simulink model "MCU_LuenbergerObserver_dsPIC33AK128MC106"  (R2024a)
settings: Solver=FixedStepDiscrete  StartTime=0.0  StopTime=inf  FixedStep=50e-6  RelTol=1e-3  EnableMultiTasking=on
undefined symbols (not defined in the file or in its folder): A0, A4, ADC, B0, C10, C11, C6, C7, C8, control, D11, D12, DiscIntNeverNeededParam, inverter, Max, MaxPer, motor, ms, NumBits1, NumBits2, P1, P17, P20, P39, P40, P41, P43, P44, P60, P61, Pin, PosRange1, PosRange2, PWM1_Trg1, Resol, s, Slope1, Slope2, us
libraries: simulink x34, MCHP_Blockset x18
(part 5 of 5)

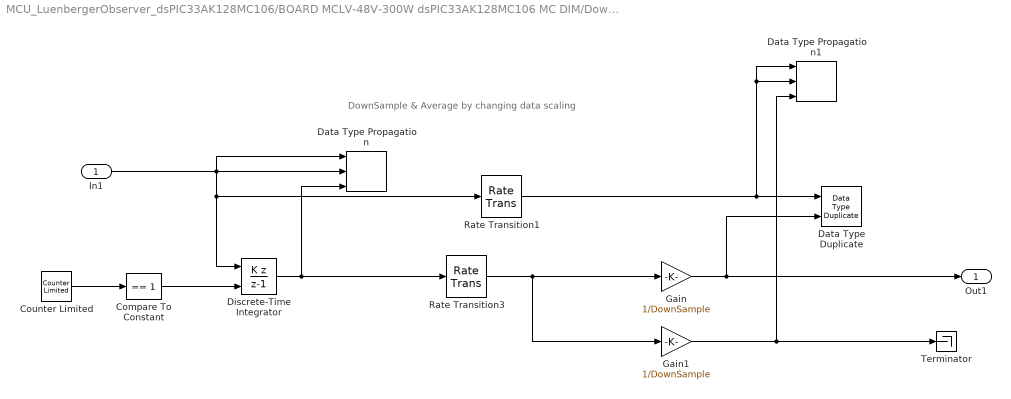
== system MCU_LuenbergerObserver_dsPIC33AK128MC106/BOARD MCLV-48V-300W dsPIC33AK128MC106 MC DIM/Downsample x20 ==
  note: DownSample & Average by changing data scaling
  In1 : Inport
  Compare To Constant : simulink/Logic and Bit Operations/Compare To Constant  relop===  const=1  OutDataTypeStr=boolean
  Counter Limited : simulink/Sources/Counter Limited  uplimit=DownSample-1  tsamp=-1
  Data Type Duplicate : DataTypeDuplicate
  Data Type Propagation : simulink/Signal Attributes/Data Type Propagation  PropDataType=fixdt(1, 16)  IfRefDouble=double  IfRefSingle=single  IsSigned=IsSigned1 or IsSigned2  NumBitsBase=NumBits1+NumBits2  NumBitsMult=1  NumBitsAdd=0  NumBitsAllowFinal=1:128  PropScaling=2^-10  ValuesUsedBestPrec=[5 -7]  SlopeBase=Slope1  SlopeMult=1  SlopeAdd=0  BiasBase=Bias1  BiasMult=1  BiasAdd=0
  Data Type Propagation1 : simulink/Signal Attributes/Data Type Propagation  PropDataType=fixdt(1, 16)  IfRefDouble=double  IfRefSingle=single  IsSigned=IsSigned1 or IsSigned2  NumBitsBase=NumBits1+NumBits2  NumBitsMult=1  NumBitsAdd=0  NumBitsAllowFinal=1:128  PropScaling=2^-10  ValuesUsedBestPrec=[5 -7]  SlopeBase=PosRange1  SlopeMult=1  SlopeAdd=0  BiasBase=Bias1  BiasMult=1  BiasAdd=0
  Discrete-Time Integrator : DiscreteIntegrator  IntegratorMethod=Accumulation: Backward Euler  gainval=1  ExternalReset=sampled level  SampleTime=-1  OutDataTypeStr=Inherit: Inherit via back propagation  ICPrevOutput=DiscIntNeverNeededParam  ICPrevScaledInput=DiscIntNeverNeededParam
  Gain : Gain  Gain=1/DownSample  OutDataTypeStr=Inherit: Inherit via back propagation  RndMeth=Round
  Gain1 : Gain  Gain=1/DownSample  OutDataTypeStr=Inherit: Inherit via back propagation
  Rate Transition1 : RateTransition  OutPortSampleTimeOpt=Multiple of input port sample time  OutPortSampleTimeMultiple=DownSample  OutPortSampleTime=DownSample
  Rate Transition3 : RateTransition  OutPortSampleTimeOpt=Multiple of input port sample time  OutPortSampleTimeMultiple=DownSample  OutPortSampleTime=DownSample
  Terminator : Terminator
  Out1 : Outport  VectorParamsAs1DForOutWhenUnconnected=off
  wires:
  Gain1/1 -> Data Type Propagation1/3, Terminator/1
  Rate Transition1/1 -> Data Type Duplicate/1, Data Type Propagation1/1, Data Type Propagation1/2
  Gain/1 -> Out1/1, Data Type Duplicate/2
  Counter Limited/1 -> Compare To Constant/1
  Discrete-Time Integrator/1 -> Rate Transition3/1, Data Type Propagation/3
  Compare To Constant/1 -> Discrete-Time Integrator/2
  In1/1 -> Data Type Propagation/1, Data Type Propagation/2, Discrete-Time Integrator/1, Rate Transition1/1
  Rate Transition3/1 -> Gain/1, Gain1/1

== system MCU_LuenbergerObserver_dsPIC33AK128MC106/BOARD MCLV-48V-300W dsPIC33AK128MC106 MC DIM/Downsample x20 _ ==
  note: DownSample & Average by changing data scaling
  In1 : Inport
  Compare To Constant : simulink/Logic and Bit Operations/Compare To Constant  relop===  const=1  OutDataTypeStr=boolean
  Counter Limited : simulink/Sources/Counter Limited  uplimit=DownSample-1  tsamp=-1
  Data Type Duplicate : DataTypeDuplicate
  Data Type Propagation : simulink/Signal Attributes/Data Type Propagation  PropDataType=fixdt(1, 16)  IfRefDouble=double  IfRefSingle=single  IsSigned=IsSigned1 or IsSigned2  NumBitsBase=NumBits1+NumBits2  NumBitsMult=1  NumBitsAdd=0  NumBitsAllowFinal=1:128  PropScaling=2^-10  ValuesUsedBestPrec=[5 -7]  SlopeBase=Slope1  SlopeMult=1  SlopeAdd=0  BiasBase=Bias1  BiasMult=1  BiasAdd=0
  Data Type Propagation1 : simulink/Signal Attributes/Data Type Propagation  PropDataType=fixdt(1, 16)  IfRefDouble=double  IfRefSingle=single  IsSigned=IsSigned1 or IsSigned2  NumBitsBase=NumBits1+NumBits2  NumBitsMult=1  NumBitsAdd=0  NumBitsAllowFinal=1:128  PropScaling=2^-10  ValuesUsedBestPrec=[5 -7]  SlopeBase=PosRange1  SlopeMult=1  SlopeAdd=0  BiasBase=Bias1  BiasMult=1  BiasAdd=0
  Discrete-Time Integrator : DiscreteIntegrator  IntegratorMethod=Accumulation: Backward Euler  gainval=1  ExternalReset=sampled level  SampleTime=-1  OutDataTypeStr=Inherit: Inherit via back propagation  ICPrevOutput=DiscIntNeverNeededParam  ICPrevScaledInput=DiscIntNeverNeededParam
  Gain : Gain  Gain=1/DownSample  OutDataTypeStr=Inherit: Inherit via back propagation  RndMeth=Round
  Gain1 : Gain  Gain=1/DownSample  OutDataTypeStr=Inherit: Inherit via back propagation
  Rate Transition1 : RateTransition  OutPortSampleTimeOpt=Multiple of input port sample time  OutPortSampleTimeMultiple=DownSample  OutPortSampleTime=DownSample
  Rate Transition3 : RateTransition  OutPortSampleTimeOpt=Multiple of input port sample time  OutPortSampleTimeMultiple=DownSample  OutPortSampleTime=DownSample
  Terminator : Terminator
  Out1 : Outport  VectorParamsAs1DForOutWhenUnconnected=off
  wires:
  Rate Transition3/1 -> Gain1/1, Gain/1
  In1/1 -> Rate Transition1/1, Discrete-Time Integrator/1, Data Type Propagation/2, Data Type Propagation/1
  Compare To Constant/1 -> Discrete-Time Integrator/2
  Discrete-Time Integrator/1 -> Data Type Propagation/3, Rate Transition3/1
  Counter Limited/1 -> Compare To Constant/1
  Gain/1 -> Data Type Duplicate/2, Out1/1
  Rate Transition1/1 -> Data Type Propagation1/2, Data Type Propagation1/1, Data Type Duplicate/1
  Gain1/1 -> Terminator/1, Data Type Propagation1/3

== system MCU_LuenbergerObserver_dsPIC33AK128MC106/BOARD MCLV-48V-300W dsPIC33AK128MC106 MC DIM/MCLV 48V-300W board webpage ==

== system MCU_LuenbergerObserver_dsPIC33AK128MC106/BOARD MCLV-48V-300W dsPIC33AK128MC106 MC DIM/Timing Analysis ==
  note: CPU overload is 0 if no overload took place between two MCU Overload block execution.
      | Otherwise, bits field output code for TID(s) responsible for at least one overload.
  Downsample Averaged2 : Subsystem  mask{InputSampleTime=.0005, DownSample=200}
      mask prompts: InputSampleTime "Input sample time"; DownSample "DownSample Factor"
  Gain : Gain  Gain=5e-9/.0005 * 100  OutMin=0  OutMax=100  OutDataTypeStr=fixdt(0,16)  RndMeth=Simplest  SaturateOnIntegerOverflow=on
  MCU Load : MCHP_Blockset/Profiling/MCU Load  MCULoadPin_TXT=None  MCULoadMeasure=on  TIMER_Resolution_TXT="Resol: 0.005(us)  -  Max: 0.328(ms)"  MCHP_TIMER_REQUEST={MCU_Load}{MCU_Load}21:5:0:0:[]:32768;  MCHP_TIMER_RESULT=[2 65535 ]  MCHP_MASTERLINK=MCU_LuenbergerObserver_dsPIC33AK128MC106/BOARD MCLV-48V-300W dsPIC33AK128MC106 MC DIM/Microchip Master  MCHP_COMPILED_INFO="CompiledSampleTime= [0.00050000000000000001041   0 ];CompiledInportDataTypes=[    ];CompiledInportDataWidth=[];"  Info="Timer 2:  Resol: 5(ns)  -  Max: 327.68(us)"  SampleTime=.0005
      settings: SourceProductName=MPLAB Device Blocks for Simulink
  MCU Overload : MCHP_Blockset/Profiling/MCU Overload  MCUOverloadBlockOutput=on  MCUOverLoadPin_TXT=None  MCHP_MASTERLINK=MCU_LuenbergerObserver_dsPIC33AK128MC106/BOARD MCLV-48V-300W dsPIC33AK128MC106 MC DIM/Microchip Master  SampleTime=-1
      settings: SourceProductName=MPLAB Device Blocks for Simulink
  Overload : Constant  Value=65535  OutDataTypeStr=Inherit: Inherit via back propagation
  Rate Transition : RateTransition  Deterministic=off  OutPortSampleTime=.0005*200
  Switch : Switch  Criteria=u2 ~= 0  SaturateOnIntegerOverflow=off  InputSameDT=off
  CPU Load : Outport  Unit=%  SampleTime=.0005*200
  CPU Overload : Outport  Port=2
  wires:
  Gain/1 -> CPU Load/1
  Overload/1 -> Switch/1
  Switch/1 -> Gain/1
  Downsample Averaged2/1(Out1) -> Switch/3
  MCU Load/1 -> Downsample Averaged2/1(In1)
  MCU Overload/1 -> CPU Overload/1, Rate Transition/1
  Rate Transition/1 -> Switch/2

== system MCU_LuenbergerObserver_dsPIC33AK128MC106/Control law/BO ==
  vdqr : Inport
  Enable : EnablePort
  vdq : Outport  VectorParamsAs1DForOutWhenUnconnected=off
  wires:
  vdqr/1 -> vdq/1

== system MCU_LuenbergerObserver_dsPIC33AK128MC106/Control law/Current Control ==
  idq : Inport
  idqr : Inport  Port=2
  om : Inport  Port=3
  gainElec : Inport  Port=4
  Enable : EnablePort  StatesWhenEnabling=reset
  Constant : Constant  Value=motor.p  OutDataTypeStr=single
  Constant1 : Constant  Value=motor.L  OutDataTypeStr=single
  Constant2 : Constant  Value=motor.Phif  OutDataTypeStr=single
  Current : Subsystem
  Voltage Saturation : Subsystem
  feedback lineazation : Subsystem
  v_dq : Outport
  wires:
  Constant1/1 -> feedback lineazation/5(L)
  Constant2/1 -> feedback lineazation/6(Phif)
  Constant/1 -> feedback lineazation/4(p)
  feedback lineazation/1(v_dq) -> Voltage Saturation/1(vdq)
  Voltage Saturation/2(saturation) -> Current/3(saturation)
  gainElec/1 -> Current/4(Ke)
  idq/1 -> Current/1(idq), feedback lineazation/2(idq)
  Current/1(v_dq) -> feedback lineazation/1(udq)
  idqr/1 -> Current/2(iqr)
  Voltage Saturation/1(vdqsat) -> v_dq/1
  om/1 -> feedback lineazation/3(om)

== system MCU_LuenbergerObserver_dsPIC33AK128MC106/Control law/Mechnical Control ==
  idqr : Inport
  om : Inport  Port=2
  omr : Inport  Port=3
  gainMeca : Inport  Port=4
  tauest : Inport  Port=5
  Enable : EnablePort  StatesWhenEnabling=reset
  Augmented state feedback : Subsystem
  Mux : Mux  Inputs=2
  Selector : Selector  InputPortWidth=2  IndexOptions=Index vector (dialog)  Indices=1  OutputSizes=1
  idqro : Outport  VectorParamsAs1DForOutWhenUnconnected=off
  wires:
  Selector/1 -> Mux/1
  Mux/1 -> idqro/1
  idqr/1 -> Selector/1
  gainMeca/1 -> Augmented state feedback/3(gainMeca)
  omr/1 -> Augmented state feedback/1(omref)
  Augmented state feedback/1(iqref) -> Mux/2
  om/1 -> Augmented state feedback/2(om)
  tauest/1 -> Augmented state feedback/4(tauest)

== system MCU_LuenbergerObserver_dsPIC33AK128MC106/Control law/Subsystem ==
  idqr : Inport
  Enable : EnablePort
  idqro : Outport
  wires:
  idqr/1 -> idqro/1

== system MCU_LuenbergerObserver_dsPIC33AK128MC106/Control law/off ==
  Enable : EnablePort
  Mux : Mux  Inputs=2
  vd : Constant  Value=0  OutDataTypeStr=single
  vq : Constant  Value=0  OutDataTypeStr=single
  vdq : Outport  VectorParamsAs1DForOutWhenUnconnected=off
  wires:
  vq/1 -> Mux/2
  Mux/1 -> vdq/1
  vd/1 -> Mux/1

== system MCU_LuenbergerObserver_dsPIC33AK128MC106/Init Enc/Wait 1s ==
  Enable : EnablePort  StatesWhenEnabling=reset
  AND : Logic  IconShape=distinctive  AllPortsSameDT=off  OutDataTypeStr=boolean
  Compare To Constant : simulink/Logic and Bit Operations/Compare To Constant  relop=>  const=0.5  OutDataTypeStr=boolean
  Compare To Constant1 : simulink/Logic and Bit Operations/Compare To Constant  relop=>  const=0.6  OutDataTypeStr=boolean
  Constant1 : Constant  OutDataTypeStr=int16
  Discrete-Time Integrator : DiscreteIntegrator  SampleTime=-1  OutDataTypeStr=fixdt(1,32,20)  SaturateOnIntegerOverflow=on  LimitOutput=on  UpperSaturationLimit=2  LowerSaturationLimit=0  ICPrevOutput=DiscIntNeverNeededParam  ICPrevScaledInput=DiscIntNeverNeededParam
  NOT : Logic  Operator=NOT  IconShape=distinctive  AllPortsSameDT=off  OutDataTypeStr=boolean
  init enc : Outport
  init done : Outport  Port=2
  wires:
  Compare To Constant/1 -> AND/1
  Constant1/1 -> Discrete-Time Integrator/1
  Discrete-Time Integrator/1 -> Compare To Constant1/1, Compare To Constant/1
  Compare To Constant1/1 -> init done/1, NOT/1
  AND/1 -> init enc/1
  NOT/1 -> AND/2

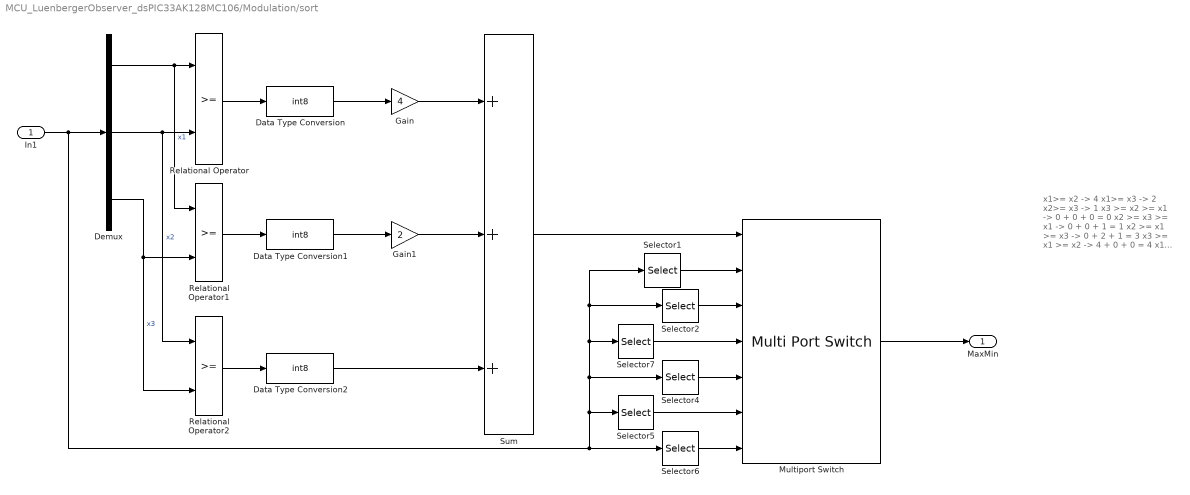
== system MCU_LuenbergerObserver_dsPIC33AK128MC106/Modulation/sort ==
  note: x1>= x2 -> 4
      | x1>= x3 -> 2
      | x2>= x3 -> 1
      |
      | x3 >= x2 >= x1 -> 0 + 0 + 0 = 0
      | x2 >= x3 >= x1 -> 0 + 0 + 1 = 1
      | x2 >= x1 >= x3 -> 0 + 2 + 1 = 3
      | x3 >= x1 >= x2 -> 4 + 0 + 0 = 4
      | x1 >= x3 >= x2 -> 4 + 2 + 0 = 6
      | x1 >= x2 >= x3 -> 4 + 2 + 1 = 7
  In1 : Inport
  Data Type Conversion : DataTypeConversion  OutDataTypeStr=int8  SaturateOnIntegerOverflow=off  RndMeth=Floor
  Data Type Conversion1 : DataTypeConversion  OutDataTypeStr=int8  SaturateOnIntegerOverflow=off  RndMeth=Floor
  Data Type Conversion2 : DataTypeConversion  OutDataTypeStr=int8  SaturateOnIntegerOverflow=off  RndMeth=Floor
  Demux : Demux  Outputs=3
  Gain : Gain  Gain=4  OutDataTypeStr=Inherit: Same as input
  Gain1 : Gain  Gain=2  OutDataTypeStr=Inherit: Same as input
  Multiport Switch : MultiPortSwitch  DataPortOrder=Specify indices  DataPortIndices={0,1,3,4,6,7}  SaturateOnIntegerOverflow=off  InputSameDT=off
  Relational Operator : RelationalOperator  OutDataTypeStr=boolean  RndMeth=Simplest  InputSameDT=off
  Relational Operator1 : RelationalOperator  OutDataTypeStr=boolean  RndMeth=Simplest  InputSameDT=off
  Relational Operator2 : RelationalOperator  OutDataTypeStr=boolean  RndMeth=Simplest  InputSameDT=off
  Selector1 : Selector  InputPortWidth=3  IndexOptions=Index vector (dialog)  Indices=[3 1]  OutputSizes=1
  Selector2 : Selector  InputPortWidth=3  IndexOptions=Index vector (dialog)  Indices=[2 1]  OutputSizes=1
  Selector4 : Selector  InputPortWidth=3  IndexOptions=Index vector (dialog)  Indices=[3 2]  OutputSizes=1
  Selector5 : Selector  InputPortWidth=3  IndexOptions=Index vector (dialog)  Indices=[1 2]  OutputSizes=1
  Selector6 : Selector  InputPortWidth=3  IndexOptions=Index vector (dialog)  Indices=[1 3]  OutputSizes=1
  Selector7 : Selector  InputPortWidth=3  IndexOptions=Index vector (dialog)  Indices=[2 3]  OutputSizes=1
  Sum : Sum  Inputs=+++
  MaxMin : Outport
  wires:
  Multiport Switch/1 -> MaxMin/1
  Selector2/1 -> Multiport Switch/3
  Selector7/1 -> Multiport Switch/4
  Selector4/1 -> Multiport Switch/5
  Selector5/1 -> Multiport Switch/6
  Selector6/1 -> Multiport Switch/7
  Selector1/1 -> Multiport Switch/2
  Sum/1 -> Multiport Switch/1
  Data Type Conversion2/1 -> Sum/3
  Gain/1 -> Sum/1
  Gain1/1 -> Sum/2
  Data Type Conversion1/1 -> Gain1/1
  Data Type Conversion/1 -> Gain/1
  Relational Operator/1 -> Data Type Conversion/1
  Relational Operator1/1 -> Data Type Conversion1/1
  Relational Operator2/1 -> Data Type Conversion2/1
  In1/1 -> Demux/1, Selector6/1, Selector5/1, Selector1/1, Selector2/1, Selector7/1, Selector4/1
  Demux/1 -> Relational Operator/1, Relational Operator1/1  "x1"
  Demux/2 -> Relational Operator/2, Relational Operator2/1  "x2"
  Demux/3 -> Relational Operator1/2, Relational Operator2/2  "x3"

== system MCU_LuenbergerObserver_dsPIC33AK128MC106/Park/Clarke ==
  note: Clark transform
      | $x_{\alpha\beta} = \frac{2}{3}\underbrace{\left[\begin{array}{ccc}1&-\frac{1}{2}&-\frac{1}{2}\\0&\frac{\sqrt{3}}{2}&-\frac{\sqrt{3}}{2}\end{array}\right]}_{C_{23}}x_{abc}$
      | if only 2 currents are measured since $x_a+x_b+x_c = 0$
      | $x_{abc} = \left[\begin{array}{cc}1 & 0\\0 & 1\\-1&-1\end{array}\right]x_{ab}$
      | leading to
      | $x_{\alpha\beta} = \underbrace{\left[\begin{array}{cc}1&0\\\frac{1}{\sqrt{3}}&\frac{2}{\sqrt{3}}\end{array}\right]}_{C_{22}}x_{ab}$
  xab(c) : Inport
  C1 : Gain  Gain=[1/sqrt(3) 2/sqrt(3)]  Multiplication=Matrix(K*u)  OutDataTypeStr=Inherit: Same as input
  Mux : Mux  Inputs=2
  Selector : Selector  InputPortWidth=2  IndexOptions=Index vector (dialog)  Indices=[1]  OutputSizes=1
  xalphabeta : Outport  VectorParamsAs1DForOutWhenUnconnected=off
  wires:
  xab(c)/1 -> Selector/1, C1/1
  Mux/1 -> xalphabeta/1
  Selector/1 -> Mux/1
  C1/1 -> Mux/2

== system MCU_LuenbergerObserver_dsPIC33AK128MC106/Park/Park ==
  note: Park
      | $x_{dq} = P(\theta)^{-1}x_{\alpha\beta}\\ P(p\theta)^{-1} = \left[\begin{array}{cc}\cos(p\theta) & \sin(p\theta)\\ -\sin(p\theta) & \cos(p\theta) \end{array}\right]$
  xalphabeta : Inport  PortDimensions=2
  P(pth) : Inport  Port=2
  Data Type Duplicate2 : DataTypeDuplicate
  Park : Product  Multiplication=Matrix(*)  OutDataTypeStr=Inherit: Inherit via back propagation  RndMeth=Round
  xdq : Outport  VectorParamsAs1DForOutWhenUnconnected=off
  wires:
  Park/1 -> Data Type Duplicate2/1, xdq/1
  xalphabeta/1 -> Data Type Duplicate2/2, Park/2
  P(pth)/1 -> Park/1

== system MCU_LuenbergerObserver_dsPIC33AK128MC106/Park inverse/Clarke Inverse ==
  note: Clarke inverse
  xalphabeta : Inport
  C23' : Gain  Gain=|  Multiplication=Matrix(K*u)  OutDataTypeStr=Inherit: Inherit via back propagation  RndMeth=Round
      | [1   -1/2        -1/2;
      |         0   sqrt(3)/2   -sqrt(3)/2]'
  xabc : Outport  VectorParamsAs1DForOutWhenUnconnected=off
  wires:
  C23'/1 -> xabc/1
  xalphabeta/1 -> C23'/1

== system MCU_LuenbergerObserver_dsPIC33AK128MC106/Park inverse/Park inverse ==
  note: Inverse Park
      | $x_{\alpha\beta} = P(p\theta)x_{dq}\\ P(p\theta) = \left[\begin{array}{cc}\cos(p\theta) & -\sin(p\theta)\\ \sin(p\theta) & \cos(p\theta) \end{array}\right]$
  xdq : Inport
  P(pth) : Inport  Port=2
  Data Type Duplicate2 : DataTypeDuplicate
  Transpose : Math  Operator=transpose
  Transpose1 : Math  Operator=transpose
  xalpha sin(pth)1 : Product  Multiplication=Matrix(*)  OutDataTypeStr=Inherit: Inherit via back propagation  RndMeth=Round
  xalpahbeta : Outport  VectorParamsAs1DForOutWhenUnconnected=off
  wires:
  xalpha sin(pth)1/1 -> Transpose1/1, Data Type Duplicate2/1
  xdq/1 -> Transpose/1
  Transpose/1 -> xalpha sin(pth)1/1, Data Type Duplicate2/2
  Transpose1/1 -> xalpahbeta/1
  P(pth)/1 -> xalpha sin(pth)1/2

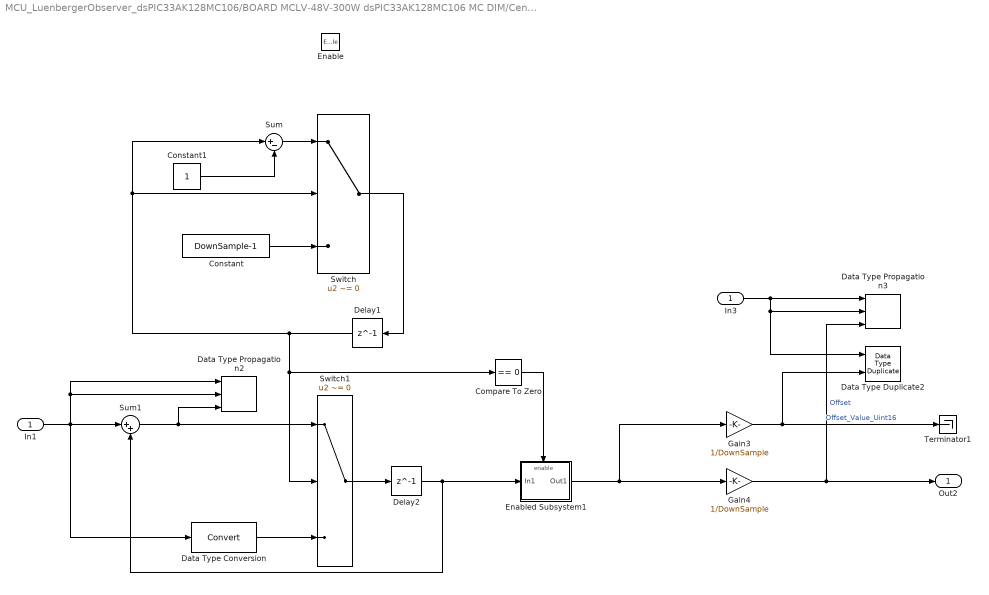
== system MCU_LuenbergerObserver_dsPIC33AK128MC106/BOARD MCLV-48V-300W dsPIC33AK128MC106 MC DIM/Center & sign reversal3/Moving Average ==
  In1 : Inport
  Enable : EnablePort  ZeroCross=off
  Compare To Zero : simulink/Logic and Bit Operations/Compare To Zero  relop===  OutDataTypeStr=boolean
  Constant : Constant  Value=DownSample-1  OutDataTypeStr=uint16
  Constant1 : Constant  OutDataTypeStr=uint16
  Data Type Duplicate2 : DataTypeDuplicate
  Data Type Propagation2 : simulink/Signal Attributes/Data Type Propagation  PropDataType=fixdt(1, 16)  IfRefDouble=double  IfRefSingle=single  IsSigned=IsSigned1 or IsSigned2  NumBitsBase=NumBits1+NumBits2  NumBitsMult=1  NumBitsAdd=0  NumBitsAllowFinal=1:128  PropScaling=2^-10  ValuesUsedBestPrec=[5 -7]  SlopeBase=Slope1  SlopeMult=1  SlopeAdd=0  BiasBase=Bias1  BiasMult=1  BiasAdd=0
  Data Type Propagation3 : simulink/Signal Attributes/Data Type Propagation  PropDataType=fixdt(1, 16)  IfRefDouble=double  IfRefSingle=single  IsSigned=IsSigned1 or IsSigned2  NumBitsBase=NumBits1+NumBits2  NumBitsMult=1  NumBitsAdd=0  NumBitsAllowFinal=1:128  PropScaling=2^-10  ValuesUsedBestPrec=[5 -7]  SlopeBase=PosRange1  SlopeMult=1  SlopeAdd=0  BiasBase=Bias1  BiasMult=1  BiasAdd=0
  Data Type Conversion : DataTypeConversion  SaturateOnIntegerOverflow=off  RndMeth=Floor
  Delay1 : Delay  DelayLength=1  InitialCondition=0
  Delay2 : Delay  DelayLength=1  InitialCondition=[InitialValue * DownSample]
  Enabled Subsystem1 : Subsystem  TreatAsAtomicUnit=on
  Gain3 : Gain  Gain=1/DownSample  OutDataTypeStr=Inherit: Inherit via back propagation  RndMeth=Round
  Gain4 : Gain  Gain=1/DownSample  OutDataTypeStr=Inherit: Inherit via back propagation
  In3 : InportShadow
  Sum : Sum  Inputs=|+-  InputSameDT=on  OutDataTypeStr=Inherit: Same as first input
  Sum1 : Sum  Inputs=|++
  Switch : Switch  Criteria=u2 ~= 0  Threshold=DownSample-1  SaturateOnIntegerOverflow=off  InputSameDT=off
  Switch1 : Switch  Criteria=u2 ~= 0  Threshold=DownSample-1  SaturateOnIntegerOverflow=off
  Terminator1 : Terminator
  Out2 : Outport  InitialOutput=[InitialValue]  VectorParamsAs1DForOutWhenUnconnected=off
  wires:
  Data Type Conversion/1 -> Switch1/3
  In3/1 -> Data Type Propagation3/1, Data Type Propagation3/2, Data Type Duplicate2/1
  Gain4/1 -> Data Type Propagation3/3, Out2/1  "Offset"
  Enabled Subsystem1/1(Out1) -> Gain3/1, Gain4/1
  Gain3/1 -> Terminator1/1, Data Type Duplicate2/2  "Offset_Value_Uint16"
  Compare To Zero/1 -> Enabled Subsystem1/Enable
  Switch1/1 -> Delay2/1
  Sum1/1 -> Switch1/1, Data Type Propagation2/3
  In1/1 -> Sum1/1, Data Type Propagation2/1, Data Type Propagation2/2, Data Type Conversion/1
  Delay2/1 -> Enabled Subsystem1/1(In1), Sum1/2
  Delay1/1 -> Compare To Zero/1, Switch1/2, Sum/1, Switch/2
  Constant/1 -> Switch/3
  Constant1/1 -> Sum/2
  Sum/1 -> Switch/1
  Switch/1 -> Delay1/1

== system MCU_LuenbergerObserver_dsPIC33AK128MC106/BOARD MCLV-48V-300W dsPIC33AK128MC106 MC DIM/Timing Analysis/Downsample Averaged2 ==
  note: DownSample & Average by changing data scaling
  In1 : Inport
  Compare To Constant : simulink/Logic and Bit Operations/Compare To Constant  relop===  const=1  OutDataTypeStr=boolean
  Counter Limited : simulink/Sources/Counter Limited  uplimit=DownSample-1  tsamp=-1
  Data Type Duplicate : DataTypeDuplicate
  Data Type Propagation : simulink/Signal Attributes/Data Type Propagation  PropDataType=fixdt(1, 16)  IfRefDouble=double  IfRefSingle=single  IsSigned=IsSigned1 or IsSigned2  NumBitsBase=NumBits1+NumBits2  NumBitsMult=1  NumBitsAdd=0  NumBitsAllowFinal=1:128  PropScaling=2^-10  ValuesUsedBestPrec=[5 -7]  SlopeBase=Slope1  SlopeMult=1  SlopeAdd=0  BiasBase=Bias1  BiasMult=1  BiasAdd=0
  Data Type Propagation1 : simulink/Signal Attributes/Data Type Propagation  PropDataType=fixdt(1, 16)  IfRefDouble=double  IfRefSingle=single  IsSigned=IsSigned1 or IsSigned2  NumBitsBase=NumBits1+NumBits2  NumBitsMult=1  NumBitsAdd=0  NumBitsAllowFinal=1:128  PropScaling=2^-10  ValuesUsedBestPrec=[5 -7]  SlopeBase=PosRange1  SlopeMult=1  SlopeAdd=0  BiasBase=Bias1  BiasMult=1  BiasAdd=0
  Discrete-Time Integrator : DiscreteIntegrator  IntegratorMethod=Accumulation: Backward Euler  gainval=1  ExternalReset=sampled level  SampleTime=-1  OutDataTypeStr=Inherit: Inherit via back propagation  ICPrevOutput=DiscIntNeverNeededParam  ICPrevScaledInput=DiscIntNeverNeededParam
  Gain : Gain  Gain=1/DownSample  OutDataTypeStr=Inherit: Inherit via back propagation
  Gain1 : Gain  Gain=1/DownSample  OutDataTypeStr=Inherit: Inherit via back propagation
  Rate Transition1 : RateTransition  Deterministic=off  OutPortSampleTime=[InputSampleTime * DownSample]
  Rate Transition3 : RateTransition  OutPortSampleTime=[InputSampleTime * DownSample]
  Terminator : Terminator
  Out1 : Outport  VectorParamsAs1DForOutWhenUnconnected=off
  wires:
  Gain1/1 -> Terminator/1, Data Type Propagation1/3
  Rate Transition1/1 -> Data Type Duplicate/1, Data Type Propagation1/1, Data Type Propagation1/2
  Gain/1 -> Out1/1, Data Type Duplicate/2
  Counter Limited/1 -> Compare To Constant/1
  Discrete-Time Integrator/1 -> Rate Transition3/1, Data Type Propagation/3
  Compare To Constant/1 -> Discrete-Time Integrator/2
  In1/1 -> Data Type Propagation/1, Data Type Propagation/2, Rate Transition1/1, Discrete-Time Integrator/1
  Rate Transition3/1 -> Gain/1, Gain1/1

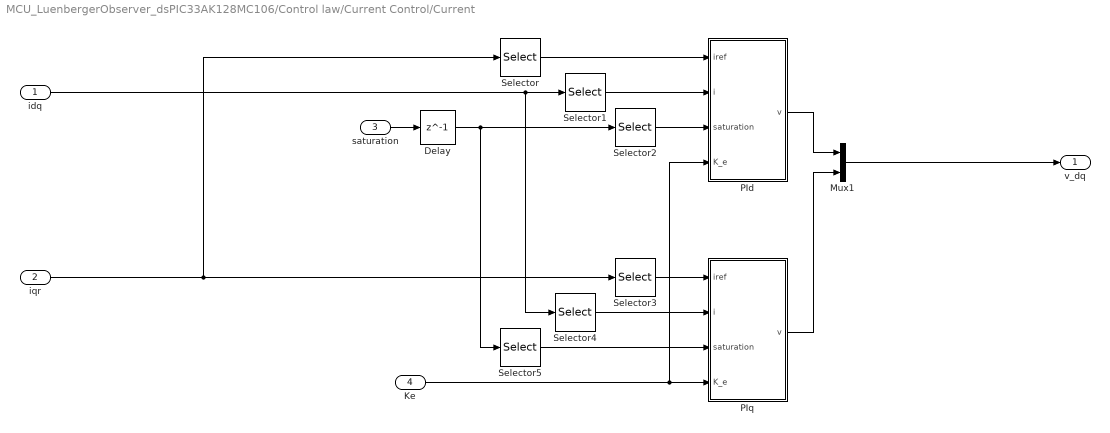
== system MCU_LuenbergerObserver_dsPIC33AK128MC106/Control law/Current Control/Current ==
  idq : Inport
  iqr : Inport  Port=2
  saturation : Inport  Port=3
  Ke : Inport  Port=4
  Delay : Delay  DelayLength=1
  Mux1 : Mux  Inputs=2
  PId : Subsystem
  PIq : Subsystem
  Selector : Selector  InputPortWidth=2  IndexOptions=Index vector (dialog)  Indices=[1]  OutputSizes=1
  Selector1 : Selector  InputPortWidth=2  IndexOptions=Index vector (dialog)  Indices=[1]  OutputSizes=1
  Selector2 : Selector  InputPortWidth=2  IndexOptions=Index vector (dialog)  Indices=[1]  OutputSizes=1
  Selector3 : Selector  InputPortWidth=2  IndexOptions=Index vector (dialog)  Indices=[2]  OutputSizes=1
  Selector4 : Selector  InputPortWidth=2  IndexOptions=Index vector (dialog)  Indices=[2]  OutputSizes=1
  Selector5 : Selector  InputPortWidth=2  IndexOptions=Index vector (dialog)  Indices=[2]  OutputSizes=1
  v_dq : Outport  VectorParamsAs1DForOutWhenUnconnected=off
  wires:
  Selector3/1 -> PIq/1(iref)
  Selector/1 -> PId/1(iref)
  iqr/1 -> Selector/1, Selector3/1
  Selector5/1 -> PIq/3(saturation)
  Selector2/1 -> PId/3(saturation)
  Delay/1 -> Selector2/1, Selector5/1
  Ke/1 -> PIq/4(K_e), PId/4(K_e)
  Mux1/1 -> v_dq/1
  Selector4/1 -> PIq/2(i)
  Selector1/1 -> PId/2(i)
  idq/1 -> Selector1/1, Selector4/1
  PId/1(v) -> Mux1/1
  PIq/1(v) -> Mux1/2
  saturation/1 -> Delay/1

== system MCU_LuenbergerObserver_dsPIC33AK128MC106/Control law/Current Control/Voltage Saturation ==
  vdq : Inport
  Divide : Product  Inputs=*/
  Gain : Gain  Gain=24/sqrt(3)
  Norm L2 : Subsystem
  Sum : Sum  Inputs=|+-
  Switch : Switch  Criteria=u2 > Threshold  Threshold=24/sqrt(3)  SaturateOnIntegerOverflow=off  InputSameDT=off
  vdqsat : Outport  VectorParamsAs1DForOutWhenUnconnected=off
  saturation : Outport  Port=2  VectorParamsAs1DForOutWhenUnconnected=off
  wires:
  Gain/1 -> Switch/1
  Norm L2/1(y) -> Divide/2, Switch/2
  Divide/1 -> Gain/1
  Switch/1 -> Sum/2, vdqsat/1
  vdq/1 -> Norm L2/1(In1), Divide/1, Sum/1, Switch/3
  Sum/1 -> saturation/1

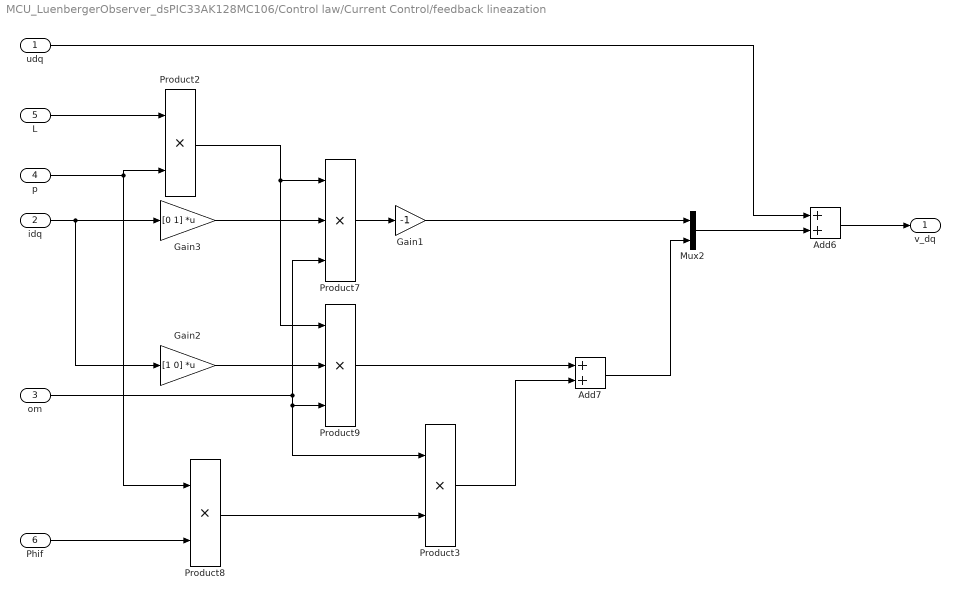
== system MCU_LuenbergerObserver_dsPIC33AK128MC106/Control law/Current Control/feedback lineazation ==
  udq : Inport
  idq : Inport  Port=2
  om : Inport  Port=3
  p : Inport  Port=4
  L : Inport  Port=5
  Phif : Inport  Port=6
  Add6 : Sum
  Add7 : Sum
  Gain1 : Gain  Gain=-1
  Gain2 : Gain  Gain=[1 0]  Multiplication=Matrix(K*u)
  Gain3 : Gain  Gain=[0 1]  Multiplication=Matrix(K*u)
  Mux2 : Mux  Inputs=2
  Product2 : Product
  Product3 : Product
  Product7 : Product  Inputs=3
  Product8 : Product
  Product9 : Product  Inputs=3
  v_dq : Outport  VectorParamsAs1DForOutWhenUnconnected=off
  wires:
  Mux2/1 -> Add6/2
  Add7/1 -> Mux2/2
  udq/1 -> Add6/1
  Add6/1 -> v_dq/1
  idq/1 -> Gain3/1, Gain2/1
  Gain1/1 -> Mux2/1
  p/1 -> Product8/1, Product2/2
  L/1 -> Product2/1
  Product2/1 -> Product9/1, Product7/1
  Gain3/1 -> Product7/2
  Product7/1 -> Gain1/1
  Phif/1 -> Product8/2
  Product8/1 -> Product3/2
  om/1 -> Product7/3, Product9/3, Product3/1
  Gain2/1 -> Product9/2
  Product9/1 -> Add7/1
  Product3/1 -> Add7/2

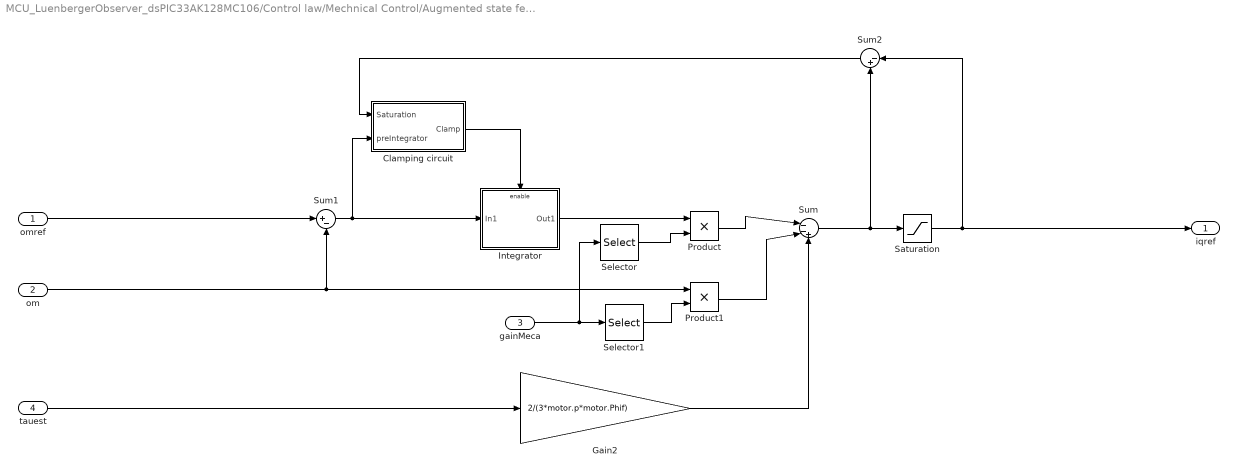
== system MCU_LuenbergerObserver_dsPIC33AK128MC106/Control law/Mechnical Control/Augmented state feedback ==
  omref : Inport
  om : Inport  Port=2
  gainMeca : Inport  Port=3
  tauest : Inport  Port=4
  Clamping circuit : Subsystem
  Gain2 : Gain  Gain=2/(3*motor.p*motor.Phif)
  Integrator : Subsystem
  Product : Product
  Product1 : Product
  Saturation : Saturate  UpperLimit=4  LowerLimit=-4
  Selector : Selector  InputPortWidth=2  IndexOptions=Index vector (dialog)  Indices=[2]  OutputSizes=1
  Selector1 : Selector  InputPortWidth=2  IndexOptions=Index vector (dialog)  Indices=1  OutputSizes=1
  Sum : Sum  Inputs=|--+  OutDataTypeStr=single  SaturateOnIntegerOverflow=on
  Sum1 : Sum  Inputs=|+-
  Sum2 : Sum  Inputs=|-+  OutDataTypeStr=Inherit: Same as accumulator  SaturateOnIntegerOverflow=on
  iqref : Outport  VectorParamsAs1DForOutWhenUnconnected=off
  wires:
  gainMeca/1 -> Selector/1, Selector1/1
  Selector/1 -> Product/2
  Selector1/1 -> Product1/2
  Saturation/1 -> iqref/1, Sum2/1
  Integrator/1(Out1) -> Product/1
  Sum2/1 -> Clamping circuit/1(Saturation)
  Clamping circuit/1(Clamp) -> Integrator/Enable
  omref/1 -> Sum1/1
  Sum1/1 -> Clamping circuit/2(preIntegrator), Integrator/1(In1)
  om/1 -> Product1/1, Sum1/2
  Product/1 -> Sum/1
  Product1/1 -> Sum/2
  Sum/1 -> Saturation/1, Sum2/2
  Gain2/1 -> Sum/3
  tauest/1 -> Gain2/1

== system MCU_LuenbergerObserver_dsPIC33AK128MC106/BOARD MCLV-48V-300W dsPIC33AK128MC106 MC DIM/Center & sign reversal3/Moving Average/Enabled Subsystem1 ==
  In1 : Inport
  Enable : EnablePort  ZeroCross=off
  Out1 : Outport
  wires:
  In1/1 -> Out1/1

== system MCU_LuenbergerObserver_dsPIC33AK128MC106/Control law/Current Control/Current/PId ==
  iref : Inport
  i : Inport  Port=2
  saturation : Inport  Port=3
  K_e : Inport  Port=4
  Clamping circuit : Subsystem
  Gain : Gain  Gain=[0 1]  Multiplication=Matrix(K*u)
  Gain1 : Gain  Gain=[1 0]  Multiplication=Matrix(K*u)
  Integrator : Subsystem
  Product : Product
  Product1 : Product
  Sum : Sum  Inputs=|--  OutDataTypeStr=single  SaturateOnIntegerOverflow=on
  Sum3 : Sum  Inputs=|+-
  v : Outport  VectorParamsAs1DForOutWhenUnconnected=off
  wires:
  saturation/1 -> Clamping circuit/2(saturation)
  Gain1/1 -> Product1/2
  Gain/1 -> Product/2
  K_e/1 -> Gain1/1, Gain/1
  Product1/1 -> Sum/2
  Product/1 -> Sum/1
  i/1 -> Product1/1, Sum3/2
  Sum3/1 -> Clamping circuit/1(preIntegrator), Integrator/1(In1)
  iref/1 -> Sum3/1
  Clamping circuit/1(Clamp) -> Integrator/Enable
  Integrator/1(Out1) -> Product/1
  Sum/1 -> v/1

== system MCU_LuenbergerObserver_dsPIC33AK128MC106/Control law/Current Control/Current/PIq ==
  iref : Inport
  i : Inport  Port=2
  saturation : Inport  Port=3
  K_e : Inport  Port=4
  Clamping circuit : Subsystem
  Gain : Gain  Gain=[0 1]  Multiplication=Matrix(K*u)
  Gain1 : Gain  Gain=[1 0]  Multiplication=Matrix(K*u)
  Integrator : Subsystem
  Product : Product
  Product1 : Product
  Sum : Sum  Inputs=|--  OutDataTypeStr=single  SaturateOnIntegerOverflow=on
  Sum3 : Sum  Inputs=|+-
  v : Outport  VectorParamsAs1DForOutWhenUnconnected=off
  wires:
  Sum/1 -> v/1
  Integrator/1(Out1) -> Product/1
  Clamping circuit/1(Clamp) -> Integrator/Enable
  iref/1 -> Sum3/1
  Sum3/1 -> Integrator/1(In1), Clamping circuit/1(preIntegrator)
  i/1 -> Sum3/2, Product1/1
  Product/1 -> Sum/1
  Product1/1 -> Sum/2
  K_e/1 -> Gain/1, Gain1/1
  Gain/1 -> Product/2
  Gain1/1 -> Product1/2
  saturation/1 -> Clamping circuit/2(saturation)

== system MCU_LuenbergerObserver_dsPIC33AK128MC106/Control law/Current Control/Voltage Saturation/Norm L2 ==
  In1 : Inport
  Dot Product : DotProduct  OutDataTypeStr=Inherit: Inherit via internal rule
  Sqrt : Sqrt
  y : Outport
  wires:
  Sqrt/1 -> y/1
  Dot Product/1 -> Sqrt/1
  In1/1 -> Dot Product/2, Dot Product/1

== system MCU_LuenbergerObserver_dsPIC33AK128MC106/Control law/Mechnical Control/Augmented state feedback/Clamping circuit ==
  note: The clamping enable or disable the integral action.
  Saturation : Inport  DisableCoverage=on
  preIntegrator : Inport  DisableCoverage=on  Port=2
  Compare To Zero1 : simulink/Logic and Bit Operations/Compare To Zero  relop=<=  OutDataTypeStr=boolean
  Delay : Delay  DelayLength=1  InitialCondition=0
  Multiply : Product
  Clamp : Outport  DisableCoverage=on  VectorParamsAs1DForOutWhenUnconnected=off
  wires:
  Compare To Zero1/1 -> Clamp/1
  preIntegrator/1 -> Multiply/2
  Multiply/1 -> Compare To Zero1/1
  Saturation/1 -> Delay/1
  Delay/1 -> Multiply/1

== system MCU_LuenbergerObserver_dsPIC33AK128MC106/Control law/Mechnical Control/Augmented state feedback/Integrator ==
  In1 : Inport
  Enable : EnablePort
  Discrete-Time Integrator : DiscreteIntegrator  SampleTime=-1  OutDataTypeStr=single  SaturateOnIntegerOverflow=on  ICPrevOutput=DiscIntNeverNeededParam  ICPrevScaledInput=DiscIntNeverNeededParam
  Out1 : Outport  VectorParamsAs1DForOutWhenUnconnected=off
  wires:
  Discrete-Time Integrator/1 -> Out1/1
  In1/1 -> Discrete-Time Integrator/1

== system MCU_LuenbergerObserver_dsPIC33AK128MC106/Control law/Current Control/Current/PId/Clamping circuit ==
  note: The clamping enable or disable the integral action.
  preIntegrator : Inport  DisableCoverage=on
  saturation : Inport  DisableCoverage=on  Port=2
  Compare To Zero1 : simulink/Logic and Bit Operations/Compare To Zero  relop=<=  OutDataTypeStr=boolean
  Multiply : Product
  Clamp : Outport  DisableCoverage=on  VectorParamsAs1DForOutWhenUnconnected=off
  wires:
  preIntegrator/1 -> Multiply/2
  Multiply/1 -> Compare To Zero1/1
  Compare To Zero1/1 -> Clamp/1
  saturation/1 -> Multiply/1

== system MCU_LuenbergerObserver_dsPIC33AK128MC106/Control law/Current Control/Current/PId/Integrator ==
  In1 : Inport
  Enable : EnablePort
  Discrete-Time Integrator : DiscreteIntegrator  SampleTime=-1  OutDataTypeStr=single  ICPrevOutput=DiscIntNeverNeededParam  ICPrevScaledInput=DiscIntNeverNeededParam
  Out1 : Outport  VectorParamsAs1DForOutWhenUnconnected=off
  wires:
  In1/1 -> Discrete-Time Integrator/1
  Discrete-Time Integrator/1 -> Out1/1

== system MCU_LuenbergerObserver_dsPIC33AK128MC106/Control law/Current Control/Current/PIq/Clamping circuit ==
  note: The clamping enable or disable the integral action.
  preIntegrator : Inport  DisableCoverage=on
  saturation : Inport  DisableCoverage=on  Port=2
  Compare To Zero1 : simulink/Logic and Bit Operations/Compare To Zero  relop=<=  OutDataTypeStr=boolean
  Multiply : Product
  Clamp : Outport  DisableCoverage=on  VectorParamsAs1DForOutWhenUnconnected=off
  wires:
  saturation/1 -> Multiply/1
  Compare To Zero1/1 -> Clamp/1
  Multiply/1 -> Compare To Zero1/1
  preIntegrator/1 -> Multiply/2

== system MCU_LuenbergerObserver_dsPIC33AK128MC106/Control law/Current Control/Current/PIq/Integrator ==
  In1 : Inport
  Enable : EnablePort
  Discrete-Time Integrator : DiscreteIntegrator  SampleTime=-1  OutDataTypeStr=single  ICPrevOutput=DiscIntNeverNeededParam  ICPrevScaledInput=DiscIntNeverNeededParam
  Out1 : Outport  VectorParamsAs1DForOutWhenUnconnected=off
  wires:
  Discrete-Time Integrator/1 -> Out1/1
  In1/1 -> Discrete-Time Integrator/1
